simulink library "library_gyro"  (Simulink 4.00)
values from neighbouring files (symbols this model uses):
  A = [0   0   0   0   1   0   0   0 ... (first row only)    [state_model_data.m]
  B = [0   0   0   0 ... (first row only)    [state_model_data.m]
  C = eye(8)    [state_model_data.m]
  D = zeros(8, 4)    [state_model_data.m]
  Omega0 = 0    [Traces_Gyros.m]
  q20 = -pi/2    (= -1.57079632679)    [Traces_Gyros.m]    (also in script_axe3_BF.m = 0; state_model_data.m = 0)
  q30 = -pi/2    (= -1.57079632679)    [Traces_Gyros.m]    (also in script_axe3_BF.m = 0; state_model_data.m = 0)
undefined symbols (not defined in the file or in its folder): K1, K2, K3, K4, Kamp, Km1, Km2, limite_ampli, OmegaMax, seuil_ampli
settings Model: LastModifiedBy=Alex

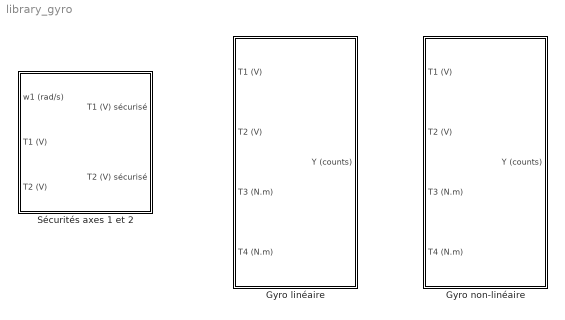
== system library_gyro ==
  Gyro linéaire : Subsystem
      settings: RTWFcnNameOpts=Auto  RTWFileNameOpts=Auto
  Gyro non-linéaire : Subsystem
      settings: RTWFcnNameOpts=Auto  RTWFileNameOpts=Auto
  Sécurités axes 1 et 2 : Subsystem
      settings: RTWFcnNameOpts=Auto  RTWFileNameOpts=Auto

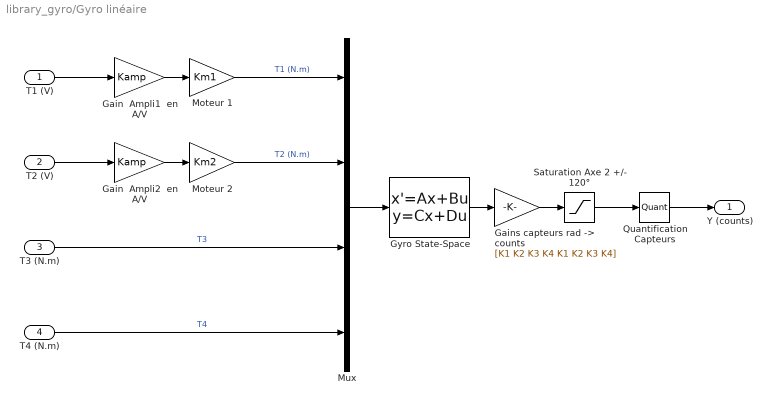
== system library_gyro/Gyro linéaire ==
  T1 (V) : Inport  Port=1  LatchInput=off
  T2 (V) : Inport  Port=2  LatchInput=off
  T3 (N.m) : Inport  Port=3  LatchInput=off
  T4 (N.m) : Inport  Port=4  LatchInput=off
  Gain  Ampli1  en A/V : Gain  Gain=Kamp  Multiplication=Element-wise(K.*u)  SaturateOnIntegerOverflow=on
  Gain  Ampli2  en A/V : Gain  Gain=Kamp  Multiplication=Element-wise(K.*u)  SaturateOnIntegerOverflow=on
  "Gains capteurs rad -> counts" : Gain  Gain=[K1 K2 K3 K4 K1 K2 K3 K4]  Multiplication=Element-wise(K.*u)  SaturateOnIntegerOverflow=on
  Gyro State-Space : StateSpace  A=A  B=B  C=C  D=D  X0=[0 q20 q30 0 Omega0 0 0 0]  AbsoluteTolerance=auto  Realization=auto
  Moteur 1 : Gain  Gain=Km1  Multiplication=Element-wise(K.*u)  SaturateOnIntegerOverflow=on
  Moteur 2 : Gain  Gain=Km2  Multiplication=Element-wise(K.*u)  SaturateOnIntegerOverflow=on
  Mux : Mux  Inputs=4
  Quantification Capteurs : Quantizer  QuantizationInterval=Q  LinearizeAsGain=on
  Saturation Axe 2 +/- 120° : Saturate  UpperLimit=[inf 120*pi/180*K2 inf inf inf inf inf inf]  LowerLimit=[-inf -120*pi/180*K2 -inf -inf -inf -inf -inf -inf]  LinearizeAsGain=on
  Y (counts) : Outport  Port=1
  wires:
  T1 (V)/1 -> Gain  Ampli1  en A/V/1
  Mux/1 -> Gyro State-Space/1
  Gain  Ampli1  en A/V/1 -> Moteur 1/1
  Moteur 2/1 -> Mux/2  "T2 (N.m)"
  Gain  Ampli2  en A/V/1 -> Moteur 2/1
  Gyro State-Space/1 -> "Gains capteurs rad -> counts"/1
  T2 (V)/1 -> Gain  Ampli2  en A/V/1
  Moteur 1/1 -> Mux/1  "T1 (N.m)"
  Saturation Axe 2 +/- 120°/1 -> Quantification Capteurs/1
  Quantification Capteurs/1 -> Y (counts)/1
  T3 (N.m)/1 -> Mux/3  "T3"
  T4 (N.m)/1 -> Mux/4  "T4"
  "Gains capteurs rad -> counts"/1 -> Saturation Axe 2 +/- 120°/1

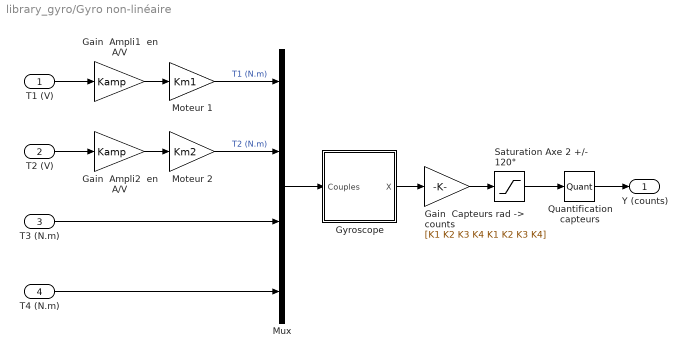
== system library_gyro/Gyro non-linéaire ==
  T1 (V) : Inport  Port=1  LatchInput=off
  T2 (V) : Inport  Port=2  LatchInput=off
  T3 (N.m) : Inport  Port=3  LatchInput=off
  T4 (N.m) : Inport  Port=4  LatchInput=off
  Gain  Ampli1  en A/V : Gain  Gain=Kamp  Multiplication=Element-wise(K.*u)  SaturateOnIntegerOverflow=on
  Gain  Ampli2  en A/V : Gain  Gain=Kamp  Multiplication=Element-wise(K.*u)  SaturateOnIntegerOverflow=on
  "Gain  Capteurs rad -> counts" : Gain  Gain=[K1 K2 K3 K4 K1 K2 K3 K4]  Multiplication=Element-wise(K.*u)  SaturateOnIntegerOverflow=on
  Gyroscope : Subsystem
      settings: RTWFcnNameOpts=Auto  RTWFileNameOpts=Auto
  Moteur 1 : Gain  Gain=Km1  Multiplication=Element-wise(K.*u)  SaturateOnIntegerOverflow=on
  Moteur 2 : Gain  Gain=Km2  Multiplication=Element-wise(K.*u)  SaturateOnIntegerOverflow=on
  Mux : Mux  Inputs=4
  Quantification capteurs : Quantizer  QuantizationInterval=Q  LinearizeAsGain=on
  Saturation Axe 2 +/- 120° : Saturate  UpperLimit=[inf 120*pi/180*K2 inf inf inf inf inf inf]  LowerLimit=[-inf -120*pi/180*K2 -inf -inf -inf -inf -inf -inf]  LinearizeAsGain=on
  Y (counts) : Outport  Port=1
  wires:
  T1 (V)/1 -> Gain  Ampli1  en A/V/1
  Mux/1 -> Gyroscope/1(Couples)
  Gain  Ampli1  en A/V/1 -> Moteur 1/1
  Moteur 2/1 -> Mux/2  "T2 (N.m)"
  Gain  Ampli2  en A/V/1 -> Moteur 2/1
  Gyroscope/1(X) -> "Gain  Capteurs rad -> counts"/1
  T2 (V)/1 -> Gain  Ampli2  en A/V/1
  Moteur 1/1 -> Mux/1  "T1 (N.m)"
  Quantification capteurs/1 -> Y (counts)/1
  T3 (N.m)/1 -> Mux/3
  T4 (N.m)/1 -> Mux/4
  "Gain  Capteurs rad -> counts"/1 -> Saturation Axe 2 +/- 120°/1
  Saturation Axe 2 +/- 120°/1 -> Quantification capteurs/1

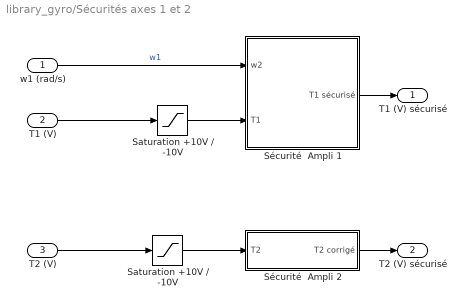
== system library_gyro/Sécurités axes 1 et 2 ==
  w1 (rad/s) : Inport  Port=1  LatchInput=off
  T1 (V) : Inport  Port=2  LatchInput=off
  T2 (V) : Inport  Port=3  LatchInput=off
  Saturation +10V / -10V : Saturate  UpperLimit=10  LowerLimit=-10  LinearizeAsGain=on
  "Saturation +10V / -10V " : Saturate  UpperLimit=10  LowerLimit=-10  LinearizeAsGain=on
  Sécurité  Ampli 1 : Subsystem
      settings: RTWFcnNameOpts=Auto  RTWFileNameOpts=Auto
  Sécurité  Ampli 2 : Subsystem
      settings: RTWFcnNameOpts=Auto  RTWFileNameOpts=Auto
  T1 (V) sécurisé : Outport  Port=1
  T2 (V) sécurisé : Outport  Port=2
  wires:
  "Saturation +10V / -10V "/1 -> Sécurité  Ampli 2/1(T2)
  w1 (rad/s)/1 -> Sécurité  Ampli 1/1(w2)  "w1"
  Saturation +10V / -10V/1 -> Sécurité  Ampli 1/2(T1)
  Sécurité  Ampli 2/1(T2 corrigé) -> T2 (V) sécurisé/1
  T2 (V)/1 -> "Saturation +10V / -10V "/1
  Sécurité  Ampli 1/1(T1 sécurisé) -> T1 (V) sécurisé/1
  T1 (V)/1 -> Saturation +10V / -10V/1

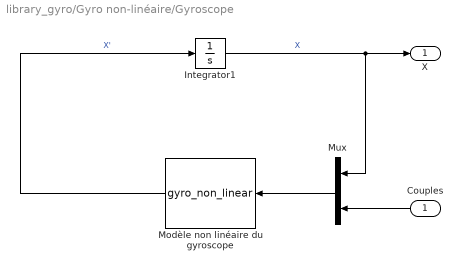
== system library_gyro/Gyro non-linéaire/Gyroscope ==
  Couples : Inport  Orientation=left  Port=1  LatchInput=off  PortDimensions=4
  Integrator1 : Integrator  ExternalReset=none  InitialConditionSource=internal  InitialCondition=[0 q20 q30 0 Omega0 0 0 0]  LimitOutput=off  UpperSaturationLimit=inf  LowerSaturationLimit=-inf  ShowSaturationPort=off  ShowStatePort=off  AbsoluteTolerance=auto
  Modèle non linéaire du gyroscope : MATLABFcn  Orientation=left  MATLABFcn=gyro_non_linear  OutputDimensions=8  OutputSignalType=auto  Output1D=on
  Mux : Mux  Orientation=left  Inputs=2
  X : Outport  Port=1
  wires:
  Modèle non linéaire du gyroscope/1 -> Integrator1/1  "X'"
  Integrator1/1 -> Mux/1, X/1  "X"
  Mux/1 -> Modèle non linéaire du gyroscope/1
  Couples/1 -> Mux/2

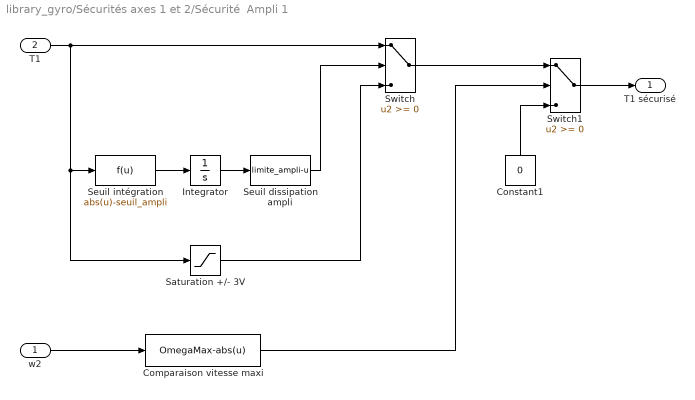
== system library_gyro/Sécurités axes 1 et 2/Sécurité  Ampli 1 ==
  w2 : Inport  Port=1  LatchInput=off
  T1 : Inport  Port=2  LatchInput=off
  Comparaison vitesse maxi : Fcn  Expr=OmegaMax-abs(u)
  Constant1 : Constant  Orientation=up  Value=0
  Integrator : Integrator  ExternalReset=none  InitialConditionSource=internal  InitialCondition=0  LimitOutput=on  UpperSaturationLimit=limite_ampli+0.1  LowerSaturationLimit=0  ShowSaturationPort=off  ShowStatePort=off  AbsoluteTolerance=auto
  Saturation +/- 3V : Saturate  UpperLimit=limite_ampli  LowerLimit=-limite_ampli  LinearizeAsGain=on
  Seuil dissipation ampli : Fcn  Expr=limite_ampli-u
  Seuil intégration : Fcn  Expr=abs(u)-seuil_ampli
  Switch : Switch  Threshold=0
  Switch1 : Switch  Threshold=0
  T1 sécurisé : Outport  Port=1
  wires:
  T1/1 -> Switch/1, Seuil intégration/1, Saturation +/- 3V/1
  Saturation +/- 3V/1 -> Switch/3
  Seuil dissipation ampli/1 -> Switch/2
  Integrator/1 -> Seuil dissipation ampli/1
  Seuil intégration/1 -> Integrator/1
  w2/1 -> Comparaison vitesse maxi/1
  Switch1/1 -> T1 sécurisé/1
  Switch/1 -> Switch1/1
  Constant1/1 -> Switch1/3
  Comparaison vitesse maxi/1 -> Switch1/2

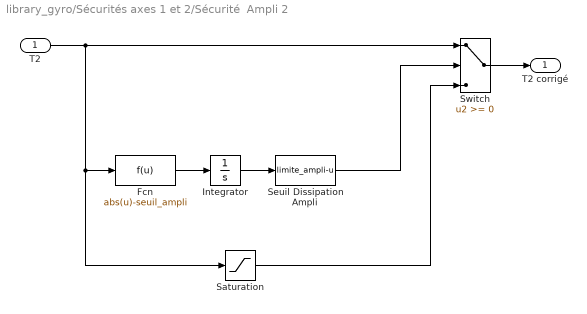
== system library_gyro/Sécurités axes 1 et 2/Sécurité  Ampli 2 ==
  T2 : Inport  Port=1  LatchInput=off
  Fcn : Fcn  Expr=abs(u)-seuil_ampli
  Integrator : Integrator  ExternalReset=none  InitialConditionSource=internal  InitialCondition=0  LimitOutput=on  UpperSaturationLimit=limite_ampli+0.1  LowerSaturationLimit=0  ShowSaturationPort=off  ShowStatePort=off  AbsoluteTolerance=auto
  Saturation : Saturate  UpperLimit=limite_ampli  LowerLimit=-limite_ampli  LinearizeAsGain=on
  Seuil Dissipation Ampli : Fcn  Expr=limite_ampli-u
  Switch : Switch  Threshold=0
  T2 corrigé : Outport  Port=1
  wires:
  T2/1 -> Switch/1, Fcn/1, Saturation/1
  Switch/1 -> T2 corrigé/1
  Seuil Dissipation Ampli/1 -> Switch/2
  Integrator/1 -> Seuil Dissipation Ampli/1
  Fcn/1 -> Integrator/1
  Saturation/1 -> Switch/3
